simulink model "simulinkmodel"  (R2021b)
settings: Solver=ode4  StartTime=0.0  StopTime=10.0  FixedStep=0.01  RelTol=1e-3
values from neighbouring files (symbols this model uses):
  B = 0.3    [parameters.m]
  D = 0.7    [parameters.m]
  J = 3.0    (= 3)    [parameters.m]
  Kd = 30    [parameters.m]
  Ki = 2.5    [parameters.m]
  Kp = 80    [parameters.m]
settings Model: Creator=Fenil  LastModifiedBy=Fenil

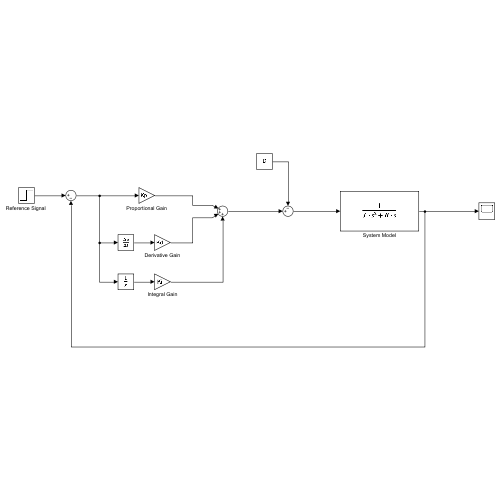
[thumbnail: Simulink's stored preview of the top-level diagram]
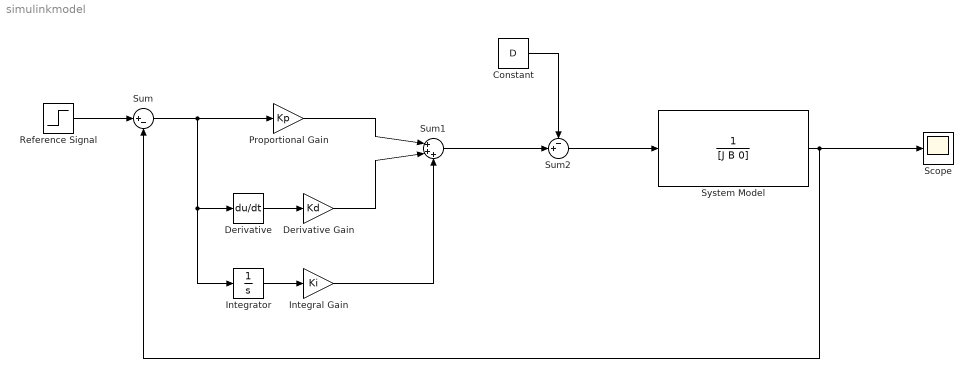
== system simulinkmodel ==
  Constant : Constant  Value=D
  Derivative : Derivative
  Derivative Gain : Gain  Gain=Kd
  Integral Gain : Gain  Gain=Ki
  Integrator : Integrator
  Proportional Gain : Gain  Gain=Kp
  "Reference Signal " : Step  SampleTime=0
  Scope : Scope
  Sum : Sum  Inputs=|+-
  Sum1 : Sum  Inputs=|+++
  Sum2 : Sum  Inputs=-+|
  System Model : TransferFcn  Denominator=[J B 0]
  wires:
  "Reference Signal "/1 -> Sum/1
  System Model/1 -> Scope/1, Sum/2
  Sum/1 -> Integrator/1, Derivative/1, Proportional Gain/1
  Derivative/1 -> Derivative Gain/1
  Derivative Gain/1 -> Sum1/2
  Proportional Gain/1 -> Sum1/1
  Sum1/1 -> Sum2/2
  Sum2/1 -> System Model/1
  Constant/1 -> Sum2/1
  Integrator/1 -> Integral Gain/1
  Integral Gain/1 -> Sum1/3
